simulink model "DFIG_1_ok_backup"  (R2022b)
settings: Solver=VariableStepAuto  StartTime=0.0  StopTime=10.0  RelTol=1e-3
InitFcn:
  | DFIG_init1
values from neighbouring files (symbols this model uses):
  D = 1e-3    (= 0.001)    [DFIG_init1.m]    (also in DFIG_init3.m; DFIG_init4.m; DFIG_init5.m; DFIG_init6.m)
  f = 50    [DFIG_init1.m]    (also in DFIG_init3.m; DFIG_init4.m; DFIG_init5.m; DFIG_init6.m)
  Fs = Vs*sqrt(2/3)/(2*pi*f)    [DFIG_init1.m]    (also in DFIG_init3.m; DFIG_init4.m; DFIG_init5.m; DFIG_init6.m)
  fsw = 4e3    (= 4000)    [DFIG_init1.m]    (also in DFIG_init3.m; DFIG_init4.m; DFIG_init5.m; DFIG_init6.m)
  J = 127    [DFIG_init1.m]    (also in DFIG_init3.m = 63.5; DFIG_init4.m = 63.5; DFIG_init5.m; DFIG_init6.m)
  ki_id = (wni^2)*Lr*sigma    (= 491.599501999)    [DFIG_init1.m]    (also in DFIG_init3.m; DFIG_init4.m; DFIG_init5.m; DFIG_init6.m = 19.6639800799)
  ki_iq = ki_id    (= 491.599501999)    [DFIG_init1.m]    (also in DFIG_init3.m; DFIG_init4.m; DFIG_init5.m; DFIG_init6.m = 19.6639800799)
  ki_n = (wnn^2)*J/p    (= 25400)    [DFIG_init1.m]    (also in DFIG_init3.m = 12700; DFIG_init4.m = 12700; DFIG_init5.m; DFIG_init6.m)
  kp_id = (2*wni*sigma*Lr)-Rr    (= 0.5771)    [DFIG_init1.m]    (also in DFIG_init3.m; DFIG_init4.m; DFIG_init5.m; DFIG_init6.m = 0.1131)
  kp_iq = kp_id    (= 0.5771)    [DFIG_init1.m]    (also in DFIG_init3.m; DFIG_init4.m; DFIG_init5.m; DFIG_init6.m = 0.1131)
  kp_n = (2*wnn*J)/p    (= 2540)    [DFIG_init1.m]    (also in DFIG_init3.m = 1270; DFIG_init4.m = 1270; DFIG_init5.m; DFIG_init6.m)
  kT = -1.5*p*(Lm/Ls)*Fs    [DFIG_init1.m]    (also in DFIG_init3.m; DFIG_init4.m; DFIG_init5.m; DFIG_init6.m)
  Lm = 2.5e-3    (= 0.0025)    [DFIG_init1.m]    (also in DFIG_init3.m; DFIG_init4.m; DFIG_init5.m; DFIG_init6.m)
  Lr = Lm + Lsi    (= 0.002587)    [DFIG_init1.m]    (also in DFIG_init3.m; DFIG_init4.m; DFIG_init5.m; DFIG_init6.m)
  Ls = Lm + Lsi    (= 0.002587)    [DFIG_init1.m]    (also in DFIG_init3.m; DFIG_init4.m; DFIG_init5.m; DFIG_init6.m)
  Lsi = 0.087e-3    (= 8.7e-05)    [DFIG_init1.m]    (also in DFIG_init3.m; DFIG_init4.m; DFIG_init5.m; DFIG_init6.m)
  p = 2    [DFIG_init1.m]    (also in DFIG_init3.m; DFIG_init4.m; DFIG_init5.m; DFIG_init6.m)
  Ps = 2e6    (= 2000000)    [DFIG_init1.m]    (also in DFIG_init3.m; DFIG_init4.m; DFIG_init5.m; DFIG_init6.m)
  Rr = 2.9e-3    (= 0.0029)    [DFIG_init1.m]    (also in DFIG_init3.m; DFIG_init4.m; DFIG_init5.m; DFIG_init6.m)
  Rs = 2.6e-3    (= 0.0026)    [DFIG_init1.m]    (also in DFIG_init3.m; DFIG_init4.m; DFIG_init5.m; DFIG_init6.m)
  sigma = 1-Lm^2/(Ls*Lr)    (= 0.0661284179513)    [DFIG_init1.m]    (also in DFIG_init3.m; DFIG_init4.m; DFIG_init5.m; DFIG_init6.m)
  Tem = 12732    [DFIG_init1.m]    (also in DFIG_init3.m; DFIG_init4.m; DFIG_init5.m; DFIG_init6.m)
  Ts = 1/fsw/50    (= 5e-06)    [DFIG_init1.m]    (also in DFIG_init3.m; DFIG_init4.m; DFIG_init5.m; DFIG_init6.m)
  Vbus = Vr_stator*sqrt(2)    [DFIG_init1.m]    (also in DFIG_init3.m; DFIG_init4.m = 1150; DFIG_init5.m = 1150; DFIG_init6.m = 1150)
  Vs = 690    [DFIG_init1.m]    (also in DFIG_init3.m; DFIG_init4.m; DFIG_init5.m; DFIG_init6.m)
undefined symbols (not defined in the file or in its folder): DiscIntNeverNeededParam
libraries: spsThreePhaseVIMeasurementLib x2, spsAsynchronousMachineSIUnitsLib x1, spsCurrentMeasurementLib x1, spsDCVoltageSourceLib x1, spsGroundLib x1, spsPWMGenerator2LevelLib x1, spsThreePhaseProgrammableVoltageSourceLib x1, spsUniversalBridgeLib x1, spsVoltageMeasurementLib x1, spspowerguiLib x1
settings Model: Creator=Qingyuan  LastModifiedBy=Qingyuan

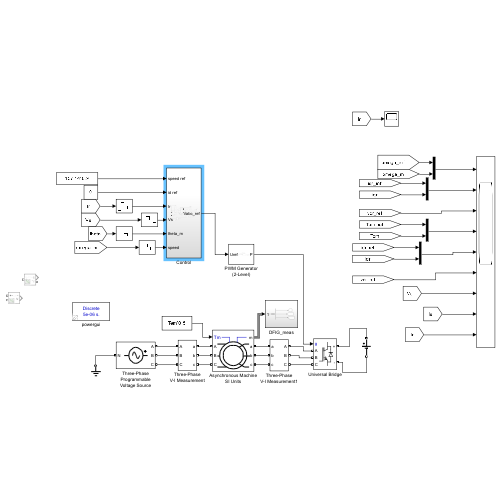
[thumbnail: Simulink's stored preview of the top-level diagram]
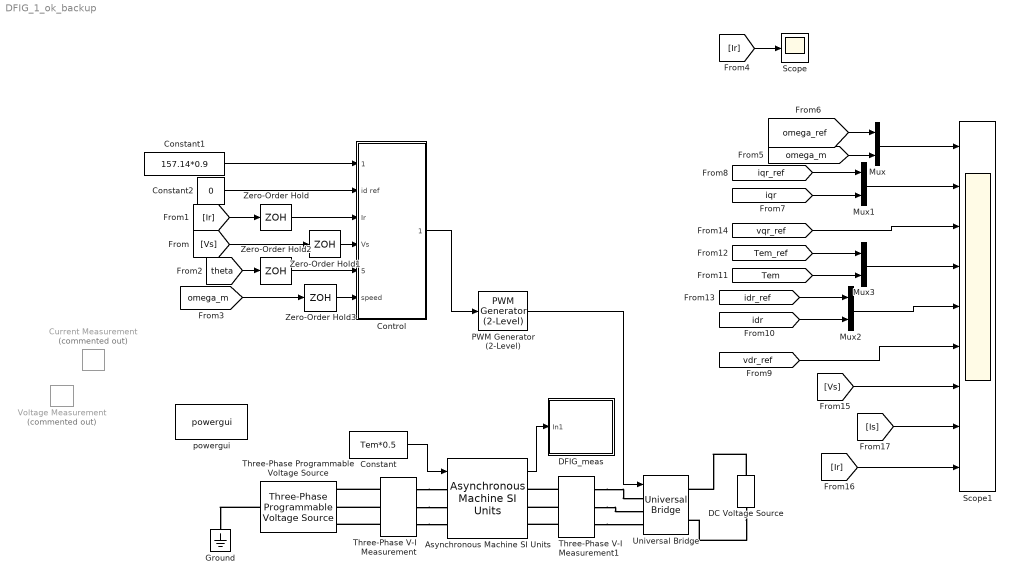
== system DFIG_1_ok_backup ==
  Asynchronous Machine SI Units : spsAsynchronousMachineSIUnitsLib/Asynchronous Machine SI Units  RotorType=Wound  PresetModel=No  MechanicalLoad=Torque Tm  ShowDetailedParameters=on  ReferenceFrame=Rotor  Units=SI  MeasurementBus=off  NominalParameters=[Ps Vs f]  VoltageRatio=1  Stator=[Rs Lsi]  Rotor=[Rr Lsi]  Cage1=[0.4155 0.002066]  Cage2=[0.4168 0.0003495]  Lm=Lm  Mechanical=[J D p]  PolePairs=2  InitialConditions=[1 0 0 0 0 0 0 0]  SimulateSaturation=off  Saturation=[14.03593122, 27.81365428, 53.79336849, 72.68890987, 97.98006896, 148.6815601, 215.7428561, 302.9841135, 428.7778367 ; 230, 322, 414, 460, 506, 552, 598, 644, 690]  LoadFlowParameters=1492000  TsPowergui=0  TsBlock=-1  IterativeModel=Trapezoidal non iterative  IterativeDiscreteModel=Trapezoidal non iterative  Pmec=1.4e6
  Constant : Constant  Value=Tem*0.5
  Constant1 : Constant  Value=157.14*0.9
  Constant2 : Constant  Value=0
  Control : Subsystem
  Current Measurement : spsCurrentMeasurementLib/Current Measurement  Commented=on  PhasorSimulation=off  OutputType=Complex  PSBequivalent=0
  DC Voltage Source : spsDCVoltageSourceLib/DC Voltage Source  Amplitude=Vbus  Measurements=None
  DFIG_meas : Subsystem
  Ground : spsGroundLib/Ground  LConnTagsString=a
  Mux{,1..3} (4 alike) : Mux  Inputs=2
  PWM Generator (2-Level) : spsPWMGenerator2LevelLib/PWM Generator (2-Level)  ModulatorType=Three-phase bridge (6 pulses)  ModulatorMode=Unsynchronized  Fc=fsw  Pc=90  nF=27  MinMax="[ -1  1 ]"  SamplingTechnique=Symmetrical regular (single edge)  ModulatingSignals=off  m=0.8  Freq=60  Phase=0  Ts=0  ShowCarrierOutport=off
  Scope : Scope
  Scope1 : Scope  NumInputPorts=9
  Three-Phase Programmable Voltage Source : spsThreePhaseProgrammableVoltageSourceLib/Three-Phase Programmable Voltage Source  PositiveSequence="[Vs  0 f]"  VariationEntity=None  VariationType=Table of time-amplitude pairs  VariationTypeAlt=Step  VariationStep=0.5  VariationRate=10  VariationMagnitude=0.3  VariationFrequency=2  VariationTiming=[1 2]  VariationPhaseA=off  Amplitudes=[1 0.8 1.2 1.0]  TimeValues=[0 0.1 0.15 0.2]  HarmonicGeneration=off  HarmonicA=[3 0.2 -25 0]  HarmonicB=[2 0.15 35 2]  Timing="[0.05  3]"  BusType=swing  Pref=0  Qref=0  Qmin=-inf  Qmax=inf
  Three-Phase V-I Measurement : spsThreePhaseVIMeasurementLib/Three-Phase V-I Measurement  VoltageMeasurement=phase-to-ground  SetLabelV=on  LabelV=Vs  Vpu=on  VpuLL=off  CurrentMeasurement=yes  SetLabelI=on  LabelI=Is  Ipu=off  Pbase=100e6  Vbase=500e3  OutputType=Complex  PhasorSimulation=off  PSBequivalent=0
  Three-Phase V-I Measurement1 : spsThreePhaseVIMeasurementLib/Three-Phase V-I Measurement  VoltageMeasurement=no  SetLabelV=off  LabelV=Vc  Vpu=off  VpuLL=off  CurrentMeasurement=yes  SetLabelI=on  LabelI=Ir  Ipu=off  Pbase=100e6  Vbase=500e3  OutputType=Complex  PhasorSimulation=off  PSBequivalent=0
  Universal Bridge : spsUniversalBridgeLib/Universal Bridge  Arms=3  SnubberResistance=1e5  SnubberCapacitance=inf  Device=IGBT / Diodes  Ron=1e-3  Lon=0  ForwardVoltages="[  0  0  ]"  ForwardVoltage=0  GTOparameters=[ 10e-6 , 20e-6 ]  IGBTparameters=[ 1e-6 , 2e-6 ]  Measurements=None  Measurements_2=None  converterType=Rectifier
  Voltage Measurement : spsVoltageMeasurementLib/Voltage Measurement  Commented=on  PhasorSimulation=off  OutputType=Complex  PSBequivalent=0
  Zero-Order Hold{,1..3} (4 alike) : ZeroOrderHold  SampleTime=1/fsw
  powergui : spspowerguiLib/powergui  Priority=1  SimulationMode=Discrete  SampleTime=Ts  frequency=60  Iterations=50  frequencyindice=50  Pbase=100e6  ErrMax=1e-4  UnitsV=kV  UnitsW=MW  buscounter=0  FunctionMessages=off  echomessages=off  EnableUseOfTLC=off  CurrentSourceSwitches=off  DisableSnubberDevices=off  DisableRonSwitches=off  DisableVfSwitches=off  DisplayEquations=off  AutomaticDiscreteSolvers=off  SolverType=Tustin/Backward Euler (TBE)  Interpol=off  ExternalGateDelay=off  methode=off  Ts=100  x0status=blocks  SPID=on  SwTol=0  HookPort=off  NonlinearTolerance=1e-4  nMaxIteration=100  ContinueOnMaxIteration=off  RestoreLinks=warning  ResistiveCurrentMeasurement=off  Frange=[0:2:500]  Ylog=off  Xlog=on  ShowGrid=off  save=off  variable=ZData  structure=0  ZoomFFT=off  StartTime=0.0  cycles=1  DisplayStyle=1  fundamental=60  FreqAxis=off  MaxFrequency=1000  frequencyindicesteady=1  RmsSteady=1  display=off
  wires:
  PWM Generator (2-Level)/1 -> Universal Bridge/1
  Control/1(Vabc_ref) -> PWM Generator (2-Level)/1
  [Vs] -> Zero-Order Hold1/1
  [Ir] -> Zero-Order Hold/1
  Constant1/1 -> Control/1(speed ref)
  Constant2/1 -> Control/2(id ref)
  [theta] -> Zero-Order Hold2/1
  [omega_m] -> Zero-Order Hold3/1
  [Ir] -> Scope/1
  [omega_ref] -> Mux/1
  [omega_m] -> Mux/2
  Mux/1 -> Scope1/1
  Mux1/1 -> Scope1/2
  [iqr] -> Mux1/2
  [iqr_ref] -> Mux1/1
  [Tem] -> Mux3/2
  Mux3/1 -> Scope1/4
  [Tem_ref] -> Mux3/1
  [idr_ref] -> Mux2/1
  [idr] -> Mux2/2
  Mux2/1 -> Scope1/5
  [Vs] -> Scope1/7
  [Ir] -> Scope1/9
  [Is] -> Scope1/8
  Asynchronous Machine SI Units/1 -> DFIG_meas/1(In1)
  Zero-Order Hold/1 -> Control/3(Ir)
  Zero-Order Hold1/1 -> Control/4(Vs)
  Zero-Order Hold2/1 -> Control/5(theta_m)
  Zero-Order Hold3/1 -> Control/6(speed)
  Constant/1 -> Asynchronous Machine SI Units/1
  [vdr_ref] -> Scope1/6
  [vqr_ref] -> Scope1/3
  connections:
  Three-Phase Programmable Voltage Source/LConn1 -- Ground/LConn1
  Three-Phase V-I Measurement/LConn1 -- Three-Phase Programmable Voltage Source/RConn1
  Three-Phase V-I Measurement/LConn2 -- Three-Phase Programmable Voltage Source/RConn2
  Three-Phase V-I Measurement/LConn3 -- Three-Phase Programmable Voltage Source/RConn3
  Three-Phase V-I Measurement/RConn1 -- Asynchronous Machine SI Units/LConn1
  Three-Phase V-I Measurement/RConn2 -- Asynchronous Machine SI Units/LConn2
  Three-Phase V-I Measurement/RConn3 -- Asynchronous Machine SI Units/LConn3
  Three-Phase V-I Measurement1/RConn1 -- Asynchronous Machine SI Units/RConn1
  Three-Phase V-I Measurement1/RConn2 -- Asynchronous Machine SI Units/RConn2
  Three-Phase V-I Measurement1/RConn3 -- Asynchronous Machine SI Units/RConn3
  Three-Phase V-I Measurement1/LConn1 -- Universal Bridge/LConn1
  Three-Phase V-I Measurement1/LConn3 -- Universal Bridge/LConn3
  Three-Phase V-I Measurement1/LConn2 -- Universal Bridge/LConn2
  DC Voltage Source/RConn1 -- Universal Bridge/RConn1
  DC Voltage Source/LConn1 -- Universal Bridge/RConn2

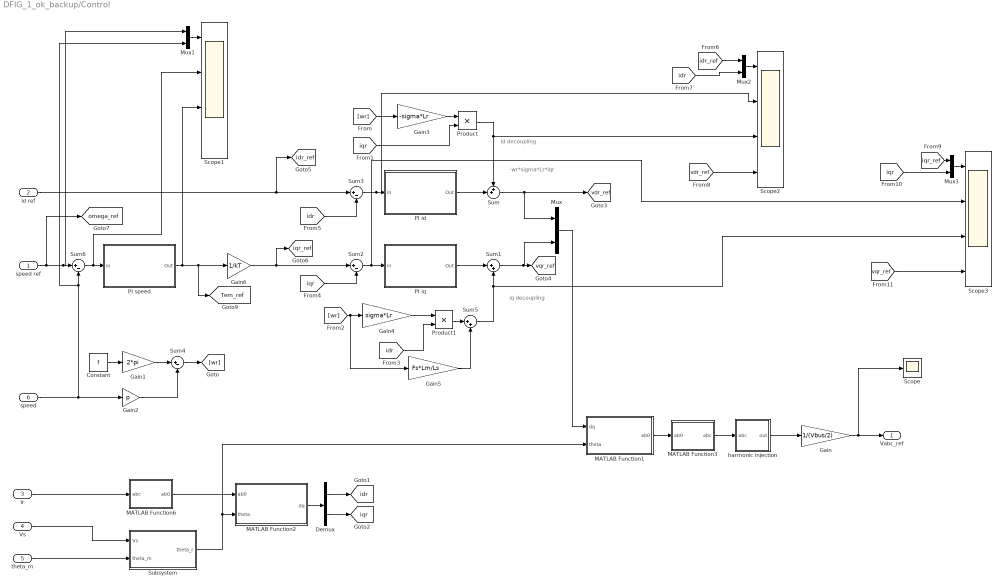
== system DFIG_1_ok_backup/Control ==
  note: -wr*sigma*Lr*iqr
  note: id decoupling
  note: iq decoupling
  speed ref : Inport
  id ref : Inport  Port=2
  Ir : Inport  Port=3
  Vs : Inport  Port=4
  theta_m : Inport  Port=5
  speed : Inport  Port=6
  Constant : Constant  Value=f
  Demux : Demux  Outputs=2
  Gain : Gain  Gain=1/(Vbus/2)
  Gain1 : Gain  Gain=2*pi
  Gain2 : Gain  Gain=p
  Gain3 : Gain  Gain=-sigma*Lr
  Gain4 : Gain  Gain=sigma*Lr
  Gain5 : Gain  Gain=Fs*Lm/Ls
  Gain6 : Gain  Gain=1/kT
  MATLAB Function1 : MATLAB Function  TreatAsAtomicUnit=on
  MATLAB Function2 : MATLAB Function  TreatAsAtomicUnit=on
  MATLAB Function3 : MATLAB Function  TreatAsAtomicUnit=on
  MATLAB Function6 : MATLAB Function  TreatAsAtomicUnit=on
  Mux{,1..3} (4 alike) : Mux  Inputs=2
  PI id : Subsystem
  PI iq : Subsystem
  PI speed : Subsystem
  Product : Product
  Product1 : Product
  Scope : Scope
  Scope1 : Scope  NumInputPorts=4
  Scope2 : Scope  NumInputPorts=4
  Scope3 : Scope  NumInputPorts=4
  Subsystem : Subsystem
  Sum : Sum  Inputs=++|
  Sum1 : Sum  Inputs=|++
  Sum{2..4,6} (4 alike) : Sum  Inputs=|+-
  Sum5 : Sum  Inputs=|++
  harmonic injection : Subsystem
  Vabc_ref : Outport
  tag scope: Tem_ref=global, idr=global, idr_ref=global, iqr=global, iqr_ref=global, omega_ref=global, vdr_ref=global, vqr_ref=global
  wires:
  MATLAB Function3/1(abc) -> harmonic injection/1(abc)
  MATLAB Function1/1(ab0) -> MATLAB Function3/1(ab0)
  Gain/1 -> Scope/1, Vabc_ref/1
  harmonic injection/1(out) -> Gain/1
  Vs/1 -> Subsystem/1(Vs)
  theta_m/1 -> Subsystem/2(theta_m)
  MATLAB Function6/1(ab0) -> MATLAB Function2/1(ab0)
  Ir/1 -> MATLAB Function6/1(abc)
  Subsystem/1(theta_r) -> MATLAB Function1/2(theta), MATLAB Function2/2(theta)
  PI iq/1(Out) -> Sum1/1
  PI id/1(Out) -> Sum/2
  Sum2/1 -> Scope3/2, PI iq/1(in)
  Sum3/1 -> Scope2/2, PI id/1(in)
  Constant/1 -> Gain1/1
  Gain1/1 -> Sum4/1
  speed/1 -> Gain2/1, Mux1/2, Sum6/2
  Gain2/1 -> Sum4/2
  Sum4/1 -> [wr]
  [wr] -> Gain3/1
  MATLAB Function2/1(dq) -> Demux/1
  Demux/2 -> [iqr]
  Demux/1 -> [idr]
  Gain3/1 -> Product/1
  [iqr] -> Product/2
  Product/1 -> Scope2/3, Sum/1
  [wr] -> Gain5/1, Gain4/1
  Gain4/1 -> Product1/1
  [idr] -> Product1/2
  Product1/1 -> Sum5/1
  Gain5/1 -> Sum5/2
  Sum5/1 -> Scope3/3, Sum1/2
  Sum/1 -> [vdr_ref], Mux/1
  Sum1/1 -> [vqr_ref], Mux/2
  Mux/1 -> MATLAB Function1/1(dq)
  Sum6/1 -> Scope1/2, PI speed/1(in)
  speed ref/1 -> [omega_ref], Mux1/1, Sum6/1
  PI speed/1(Out) -> Scope1/3, [Tem_ref], Gain6/1
  id ref/1 -> [idr_ref], Sum3/1
  Gain6/1 -> [iqr_ref], Sum2/1
  [iqr] -> Sum2/2
  [idr] -> Sum3/2
  Mux1/1 -> Scope1/1
  Mux2/1 -> Scope2/1
  [idr_ref] -> Mux2/1
  [idr] -> Mux2/2
  [vdr_ref] -> Scope2/4
  Mux3/1 -> Scope3/1
  [iqr_ref] -> Mux3/1
  [iqr] -> Mux3/2
  [vqr_ref] -> Scope3/4

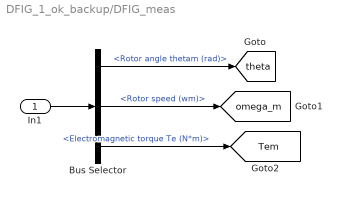
== system DFIG_1_ok_backup/DFIG_meas ==
  In1 : Inport
  Bus Selector : BusSelector  OutputSignals=Mechanical.Rotor angle thetam (rad),Mechanical.Rotor speed (wm),Mechanical.Electromagnetic torque Te (N*m)
  tag scope: Tem=global, omega_m=global, theta=global
  wires:
  Bus Selector/1 -> [theta]  "<Rotor angle thetam (rad)>"
  Bus Selector/2 -> [omega_m]  "<Rotor speed (wm)>"
  In1/1 -> Bus Selector/1
  Bus Selector/3 -> [Tem]  "<Electromagnetic torque Te (N*m)>"

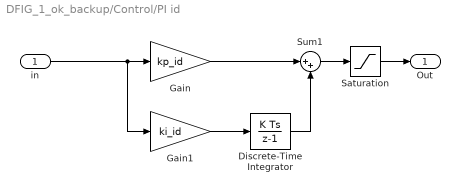
== system DFIG_1_ok_backup/Control/PI id ==
  in : Inport
  Discrete-Time Integrator : DiscreteIntegrator  SampleTime=1/fsw  LimitOutput=on  UpperSaturationLimit=Vbus/sqrt(3)  LowerSaturationLimit=-Vbus/sqrt(3)  ICPrevOutput=DiscIntNeverNeededParam  ICPrevScaledInput=DiscIntNeverNeededParam
  Gain : Gain  Gain=kp_id
  Gain1 : Gain  Gain=ki_id
  Saturation : Saturate  UpperLimit=Vbus/sqrt(3)  LowerLimit=-Vbus/sqrt(3)
  Sum1 : Sum  Inputs=|++
  Out : Outport
  wires:
  in/1 -> Gain1/1, Gain/1
  Gain1/1 -> Discrete-Time Integrator/1
  Gain/1 -> Sum1/1
  Discrete-Time Integrator/1 -> Sum1/2
  Sum1/1 -> Saturation/1
  Saturation/1 -> Out/1

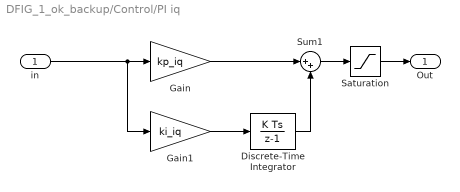
== system DFIG_1_ok_backup/Control/PI iq ==
  in : Inport
  Discrete-Time Integrator : DiscreteIntegrator  SampleTime=1/fsw  LimitOutput=on  UpperSaturationLimit=Vbus/sqrt(3)  LowerSaturationLimit=-Vbus/sqrt(3)  ICPrevOutput=DiscIntNeverNeededParam  ICPrevScaledInput=DiscIntNeverNeededParam
  Gain : Gain  Gain=kp_iq
  Gain1 : Gain  Gain=ki_iq
  Saturation : Saturate  UpperLimit=Vbus/sqrt(3)  LowerLimit=-Vbus/sqrt(3)
  Sum1 : Sum  Inputs=|++
  Out : Outport
  wires:
  Saturation/1 -> Out/1
  Sum1/1 -> Saturation/1
  Discrete-Time Integrator/1 -> Sum1/2
  Gain/1 -> Sum1/1
  Gain1/1 -> Discrete-Time Integrator/1
  in/1 -> Gain/1, Gain1/1

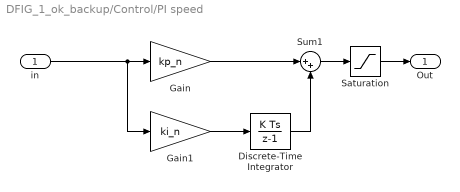
== system DFIG_1_ok_backup/Control/PI speed ==
  in : Inport
  Discrete-Time Integrator : DiscreteIntegrator  SampleTime=1/fsw  LimitOutput=on  UpperSaturationLimit=Tem  LowerSaturationLimit=-Tem  ICPrevOutput=DiscIntNeverNeededParam  ICPrevScaledInput=DiscIntNeverNeededParam
  Gain : Gain  Gain=kp_n
  Gain1 : Gain  Gain=ki_n
  Saturation : Saturate  UpperLimit=Tem  LowerLimit=-Tem
  Sum1 : Sum  Inputs=|++
  Out : Outport
  wires:
  Saturation/1 -> Out/1
  Sum1/1 -> Saturation/1
  Discrete-Time Integrator/1 -> Sum1/2
  Gain/1 -> Sum1/1
  Gain1/1 -> Discrete-Time Integrator/1
  in/1 -> Gain/1, Gain1/1

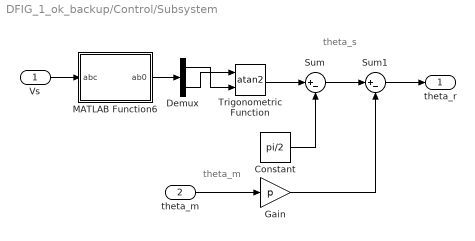
== system DFIG_1_ok_backup/Control/Subsystem ==
  note: theta_s
  note: theta_m
  Vs : Inport
  theta_m : Inport  Port=2
  Constant : Constant  Value=pi/2
  Demux : Demux  Outputs=2
  Gain : Gain  Gain=p
  MATLAB Function6 : MATLAB Function  TreatAsAtomicUnit=on
  Sum : Sum  Inputs=|+-
  Sum1 : Sum  Inputs=|+-
  Trigonometric Function : Trigonometry  Operator=atan2
  theta_r : Outport
  wires:
  Vs/1 -> MATLAB Function6/1(abc)
  theta_m/1 -> Gain/1
  MATLAB Function6/1(ab0) -> Demux/1
  Demux/1 -> Trigonometric Function/2
  Demux/2 -> Trigonometric Function/1
  Trigonometric Function/1 -> Sum/1
  Constant/1 -> Sum/2
  Sum/1 -> Sum1/1
  Sum1/1 -> theta_r/1
  Gain/1 -> Sum1/2

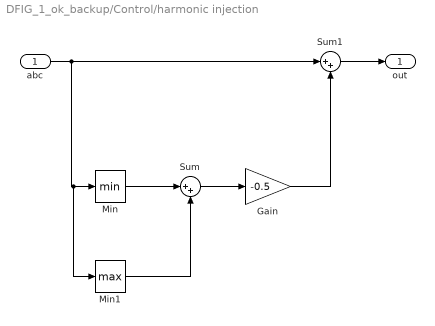
== system DFIG_1_ok_backup/Control/harmonic injection ==
  abc : Inport
  Gain : Gain  Gain=-0.5
  Min : MinMax
  Min1 : MinMax  Function=max
  Sum : Sum  Inputs=|++
  Sum1 : Sum  Inputs=|++
  out : Outport
  wires:
  Min/1 -> Sum/1
  Min1/1 -> Sum/2
  Sum1/1 -> out/1
  Sum/1 -> Gain/1
  abc/1 -> Min1/1, Min/1, Sum1/1
  Gain/1 -> Sum1/2

== matlab function DFIG_1_ok_backup/Control/MATLAB Function3 ==
  data: ab0 input; abc output
function abc = ab0_to_abc(ab0)
abc = zeros(3,1);
abc(1) = ab0(1);
abc(2) = -1/2 * ab0(1) + sqrt(3)/2 * ab0(2);
abc(3) = -1/2 * ab0(1) - sqrt(3)/2 * ab0(2);
end

== matlab function DFIG_1_ok_backup/Control/Subsystem/MATLAB Function6 ==
  data: abc input; ab0 output
function ab0 = abc_to_ab0(abc)
ab0 = zeros(2,1);
ab0(1) = 2/3 * (abc(1) - abc(2)/2 - abc(3)/2);
ab0(2) = 2/3 * ( (sqrt(3)/2)*abc(2) - (sqrt(3)/2)*abc(3));
end

== matlab function DFIG_1_ok_backup/Control/MATLAB Function2 ==
  data: ab0 input; dq output; theta input
function dq = ab0_to_dq(ab0, theta)
dq = zeros(2,1);
dq(1) = cos(theta)*ab0(1) + sin(theta)*ab0(2);
dq(2) = -sin(theta)*ab0(1) + cos(theta)*ab0(2);
end

== matlab function DFIG_1_ok_backup/Control/MATLAB Function6 ==
  data: abc input; ab0 output
function ab0 = abc_to_ab0(abc)
ab0 = zeros(2,1);
ab0(1) = 2/3 * (abc(1) - abc(2)/2 - abc(3)/2);
ab0(2) = 2/3 * ( (sqrt(3)/2)*abc(2) - (sqrt(3)/2)*abc(3));
end

== matlab function DFIG_1_ok_backup/Control/MATLAB Function1 ==
  data: dq input; ab0 output; theta input
function ab0 = dq_to_ab0(dq, theta)
ab0 = zeros(2,1);
ab0(1) = dq(1) * cos(theta) - dq(2) * sin(theta);
ab0(2) = dq(1) * sin(theta) + dq(2) * cos(theta);

end
